simulink model "filtrage_Simulink__moving_average"  (R2019b)
settings: Solver=VariableStepAuto  StartTime=0.0  StopTime=10.0  RelTol=1e-3
InitFcn:
  | load filtrage_pb_ordre_1.mat;
libraries: dspstat3 x1
settings Model: Creator=ivanl  LastModifiedBy=ivanl

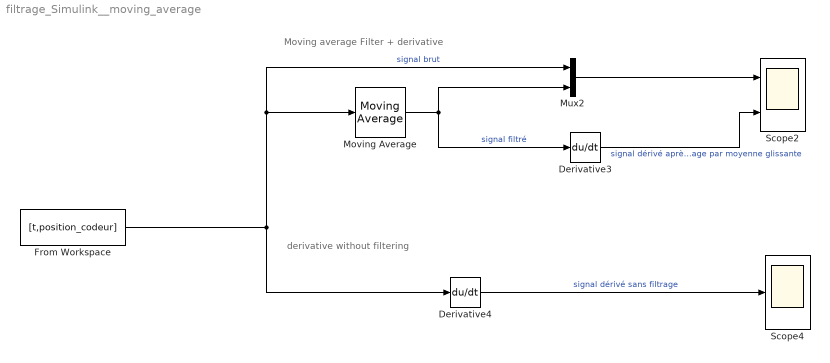
== system filtrage_Simulink__moving_average ==
  note: derivative without filtering
  note: Moving average Filter + derivative
  Derivative3 : Derivative
  Derivative4 : Derivative
  From Workspace : FromWorkspace  VariableName=[t,position_codeur]  SampleTime=0.001
  Moving Average : dspstat3/Moving Average  Method=Sliding window  ForgettingFactorPort=off  SpecifyWindowLength=on  WindowLength=300  ForgettingFactor=0.9  SimulateUsing=Code generation
  Mux2 : Mux  Inputs=2
  Scope2 : Scope  NumInputPorts=2
  Scope4 : Scope
  wires:
  Moving Average/1 -> Mux2/2, Derivative3/1  "signal filtré"
  Derivative3/1 -> Scope2/2  "signal dérivé après filtrage par moyenne glissante"
  Mux2/1 -> Scope2/1
  Derivative4/1 -> Scope4/1  "signal dérivé sans filtrage"
  From Workspace/1 -> Derivative4/1, Moving Average/1, Mux2/1  "signal brut"
